simulink model "SinusoidalStimulation"  (R2012b)
settings: Solver=ode1  StartTime=0.0  StopTime=tend+3  FixedStep=0.001  RelTol=1e-3
undefined symbols (not defined in the file): F1, F2, F3, HIL, LCconv, sat, thresh, U1, U2
libraries: quarc_library x4, ScienceStimHasomed_Lib x1, simulink x1
settings Model: SimulationMode=external  ExtModeTrigDuration=5000000  Creator=LabUser  LastModifiedBy=LabUser
settings SolverCC: PositivePriorityOrder=on
settings DataIOCC: LimitDataPoints=off
settings DebuggingCC: SolverPrmCheckMsg=none
settings RTWCC: SystemTargetFile=quarc_win64.tlc  TemplateMakefile=quarc_default_tmf  Description=QUARC Win64 Target  ProcessScript=quarc_win64_make_rtw_hook
settings RTWCC: CustomLibrary=|
  | sciencemode.obj
  | serial_windows.obj
settings STFCustomTargetCC: TargetPreCompLibLocation=C:\PROGRA~3\QUARC\lib\2012b\win64\release  CodeReplacementLibrary=ANSI_C  GeneratePreprocessorConditionals=Disable all  CombineOutputUpdateFcns=on  GRTInterface=off  SystemTargetFile=quarc_win64.tlc
settings GRTTargetCC: TargetPreCompLibLocation=C:\PROGRA~3\QUARC\lib\2012b\win64\release  ParMdlRefBuildCompliant=off  CompOptLevelCompliant=off  ConcurrentExecutionCompliant=off  MatFileLogging=off  ExtMode=on  ExtModeMexFile=quarc_comm

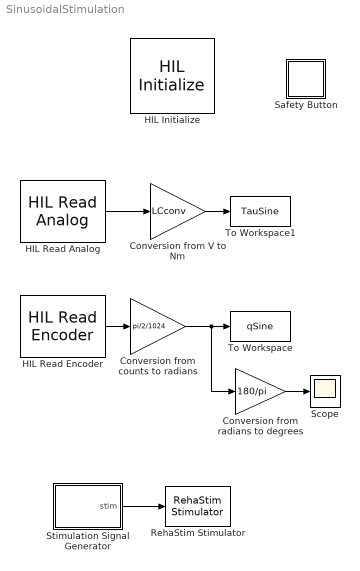
== system SinusoidalStimulation ==
  Conversion from V to Nm : Gain  Gain=LCconv
  Conversion from counts to radians : Gain  Gain=pi/2/1024
  Conversion from radians to degrees : Gain  Gain=180/pi
  HIL Initialize : quarc_library/Data Acquisition/Generic/Configuration/HIL Initialize  Priority=-99  object_name=HIL-1  board_type=qpid_e  board_number=0  board_options=enc0_dir=0;enc0_filter=1;enc0_a=1;enc0_b=1;enc0_z=0;enc0_reload=0;enc1_dir=0;enc1_filter=1;enc1_a=1;enc1_b=1;enc1_z=0;enc1_reload=0;enc2_dir=0;enc2_filter=1;enc2_a=1;enc2_b=1;enc2_z=0;enc2_reload=0;enc3_dir=0;enc3_filter=1;enc3_a=1;enc3_b=1;enc3_z=0;enc3_reload=0;enc4_dir=0;enc4_filter=1;enc4_a=1;enc4_b=1;enc4_z=0;enc4_reload=0;enc5_dir=0;enc5_filter=1;enc5_a=1;enc5_b=1;enc5_z=0;enc5_reload=0;enc6_dir=0;enc6_filter=1;enc6_a=1;enc6_b=1;enc6_z=0;enc6_reload=0;enc7_dir=0;enc7_filter=1;enc7_a=1;enc7_b=1;enc7_z=0;enc7_reload=0;ext_int_polarity=0;fuse_polarity=0;convert_polarity=0;watchdog_polarity=0;ext_int_watchdog=0;fuse_watchdog=0;trig1_watchdog=0;watchdog_to_trig1=0;watchdog_to_trig2=0;counter_to_trig0=0;trigger_adcs=0;latch_on_adc=0;pwm_immediate=0  exclusive=off  active=off  hardware_clocks=[0:16]  clock_modes=[]  initial_clock_frequencies=[]  set_clock_params_at_start=off  set_clock_params_at_switch_in=off  set_clock_frequencies_at_start=off  set_clock_frequencies_at_switch_in=off  analog_input_channels=[0:7]  analog_input_maximums=10  analog_input_minimums=-10  set_analog_input_params_at_start=off  set_analog_input_params_at_switch_in=off  analog_output_channels=[0:7]  analog_output_maximums=10  analog_output_minimums=-10  initial_analog_outputs=[0]  final_analog_outputs=[0]  watchdog_analog_outputs=0  set_analog_output_params_at_start=off  set_analog_output_params_at_switch_in=off  set_analog_outputs_at_start=on  set_analog_outputs_at_switch_in=off  set_analog_outputs_at_terminate=on  set_analog_outputs_at_switch_out=off  set_analog_outputs_on_watchdog=off  digital_input_channels=[]  digital_output_channels=[]  digital_output_configuration=[]  initial_digital_outputs=[1]  final_digital_outputs=[1]  watchdog_digital_outputs=[2]  set_digital_output_params_at_start=off  set_digital_output_params_at_switch_in=off  set_digital_outputs_at_start=on  set_digital_outputs_at_switch_in=off  set_digital_outputs_at_terminate=on  set_digital_outputs_at_switch_out=off  set_digital_outputs_on_watchdog=off  encoder_channels=[0:7]  quadrature=[4]  encoder_filter_frequency=40e6/1  initial_encoder_counts=[0]  set_encoder_params_at_start=on  set_encoder_params_at_switch_in=off  set_encoder_counts_at_start=off  set_encoder_counts_at_switch_in=off  pwm_channels=[0:7]  pwm_modes=0  pwm_frequency=40e6/4096  pwm_configuration=[0]  pwm_alignment=[0]  pwm_polarity=[1]  pwm_leading_deadband=[0]  pwm_trailing_deadband=[0]  initial_pwm_outputs=[0]  final_pwm_outputs=[0]  watchdog_pwm_outputs=[0]  set_pwm_params_at_start=on  set_pwm_params_at_switch_in=off  set_pwm_outputs_at_start=on  set_pwm_outputs_at_switch_in=off  set_pwm_outputs_at_terminate=on  set_pwm_outputs_at_switch_out=off  set_pwm_outputs_on_watchdog=off  other_output_channels=[]  initial_other_outputs=[]  final_other_outputs=[]  watchdog_other_outputs=[]  set_other_outputs_at_start=off  set_other_outputs_at_switch_in=off  set_other_outputs_at_terminate=off  set_other_outputs_at_switch_out=off  set_other_outputs_on_watchdog=off
  HIL Read Analog : quarc_library/Data Acquisition/Generic/Immediate I//O/HIL Read Analog  object_name=HIL-1  channels=0  sample_time=qc_get_step_size  active=on  vector_output=off
  HIL Read Encoder : quarc_library/Data Acquisition/Generic/Immediate I//O/HIL Read Encoder  object_name=HIL-1  channels=0  sample_time=qc_get_step_size  active=on  vector_output=off  data_type_mode=Inherit via back propagation  data_type=double
  RehaStim Stimulator : ScienceStimHasomed_Lib/RehaStim Stimulator  sFreq=1000  Freq=stimfreq  PWidth=PW
  Safety Button : Subsystem
  Scope : Scope
      settings: YMin=0  YMax=90
  Stimulation Signal Generator : Subsystem  mask{F1=F1, F2=F2, F3=F3, U1=U1, U2=U2}
      mask prompts: F1 "First frequency [Hz]:"; F2 "Second frequency [Hz]:"; F3 "Third frequency [Hz]:"; U1 "Minimum normalized stimulation ampiltude:"; U2 "Maximum normalized stimulation ampiltude:"
  To Workspace : ToWorkspace  VariableName=qSine  SampleTime=-1
  To Workspace1 : ToWorkspace  VariableName=TauSine  SampleTime=-1
  wires:
  Conversion from counts to radians/1 -> Conversion from radians to degrees/1, To Workspace/1
  Stimulation Signal Generator/1("stim ") -> RehaStim Stimulator/1
  HIL Read Encoder/1 -> Conversion from counts to radians/1
  Conversion from radians to degrees/1 -> Scope/1
  HIL Read Analog/1 -> Conversion from V to Nm/1
  Conversion from V to Nm/1 -> To Workspace1/1

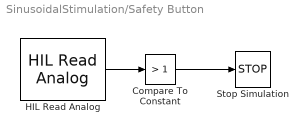
== system SinusoidalStimulation/Safety Button ==
  Compare To Constant : simulink/Logic and Bit Operations/Compare To Constant  relop=>  const=1  OutDataTypeStr=boolean
  HIL Read Analog : quarc_library/Data Acquisition/Generic/Immediate I//O/HIL Read Analog  object_name=HIL-1  channels=[7]  sample_time=qc_get_step_size  active=on  vector_output=off
  Stop Simulation : Stop
  wires:
  HIL Read Analog/1 -> Compare To Constant/1
  Compare To Constant/1 -> Stop Simulation/1

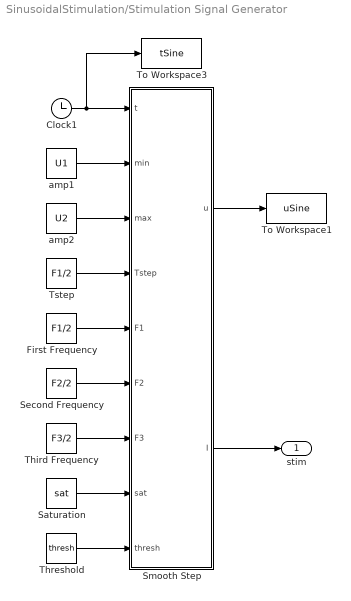
== system SinusoidalStimulation/Stimulation Signal Generator ==
  Clock1 : Clock
  First Frequency : Constant  Value=F1/2
  Saturation : Constant  Value=sat
  Second Frequency : Constant  Value=F2/2
  Smooth Step : MATLAB Function  TreatAsAtomicUnit=on
  Third Frequency : Constant  Value=F3/2
  Threshold : Constant  Value=thresh
  To Workspace1 : ToWorkspace  VariableName=uSine  SampleTime=-1
  To Workspace3 : ToWorkspace  VariableName=tSine  SampleTime=-1
  Tstep : Constant  Value=F1/2
  amp1 : Constant  Value=U1
  amp2 : Constant  Value=U2
  "stim " : Outport
  wires:
  Clock1/1 -> To Workspace3/1, Smooth Step/1(t)
  amp1/1 -> Smooth Step/2(min)
  Tstep/1 -> Smooth Step/4(Tstep)
  amp2/1 -> Smooth Step/3(max)
  First Frequency/1 -> Smooth Step/5(F1)
  Second Frequency/1 -> Smooth Step/6(F2)
  Third Frequency/1 -> Smooth Step/7(F3)
  Saturation/1 -> Smooth Step/8(sat)
  Threshold/1 -> Smooth Step/9(thresh)
  Smooth Step/2(I) -> "stim "/1
  Smooth Step/1(u) -> To Workspace1/1

== matlab function SinusoidalStimulation/Stimulation Signal Generator/Smooth Step ==
  data: t input; min input; max input; u output; Tstep input; F1 input; F2 input; F3 input; sat input; thresh input; I output
function [u,I] = fcn(t,min,max,Tstep,F1,F2,F3,sat,thresh)

amp1 = max/2;
amp2 = (max-min)/2;
tend = 8*F1;

if (t < tend)
    if t < Tstep
        u = amp1*(1-cos(t*pi/Tstep));
    elseif (t >= Tstep) && (t < Tstep+4*F1)
        u = amp1+(amp1-amp2)+amp2*cos((t-Tstep)*pi/F1);
    elseif (t >= Tstep+4*F1) && (t < Tstep+4*F1+4*F2)
        u = amp1+(amp1-amp2)+amp2*cos((t-(Tstep+4*F1))*pi/F2);
    elseif (t >= Tstep+4*F1+4*F2) && (t < tend)
        u = amp1+(amp1-amp2)+amp2*cos((t-(Tstep+4*F1+4*F2))*pi/F3);
    else
        u = 0;
    end
    
    I = thresh+u*(sat-thresh);
    
else
    u = 0;
    I = 0;
end
